simulink model "ICare_Simulink_Demo"  (R2026a)
settings: Solver=FixedStepDiscrete  StopTime=0
settings Model: Creator=ragav  LastModifiedBy=ragav

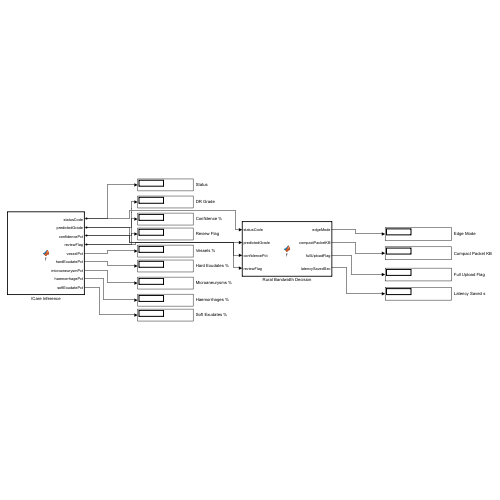
[thumbnail: Simulink's stored preview of the top-level diagram]
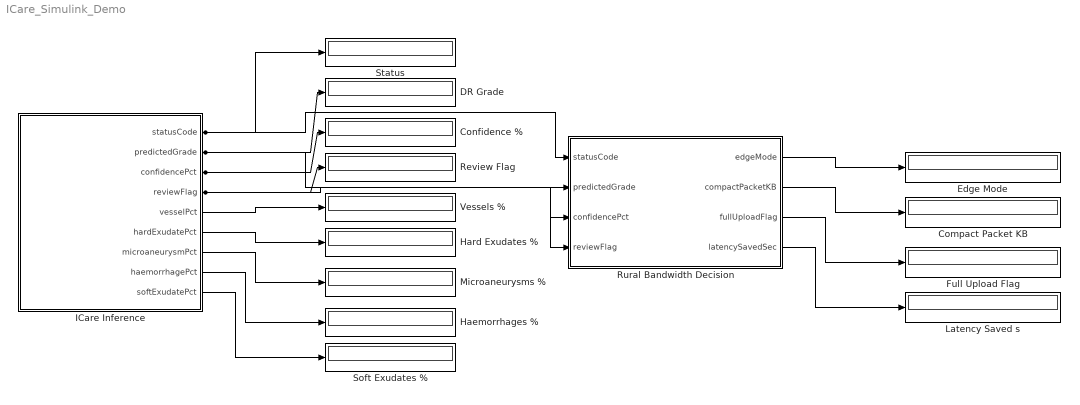
== system ICare_Simulink_Demo ==
  Compact Packet KB : Display
  Confidence % : Display
  DR Grade : Display
  Edge Mode : Display
  Full Upload Flag : Display
  Haemorrhages % : Display
  Hard Exudates % : Display
  ICare Inference : MATLAB Function  TreatAsAtomicUnit=on
  Latency Saved s : Display
  Microaneurysms % : Display
  Review Flag : Display
  Rural Bandwidth Decision : MATLAB Function  TreatAsAtomicUnit=on
  Soft Exudates % : Display
  Status : Display
  Vessels % : Display
  wires:
  ICare Inference/1(statusCode) -> Status/1, Rural Bandwidth Decision/1(statusCode)
  ICare Inference/2(predictedGrade) -> DR Grade/1, Rural Bandwidth Decision/2(predictedGrade)
  ICare Inference/3(confidencePct) -> Confidence %/1, Rural Bandwidth Decision/3(confidencePct)
  ICare Inference/4(reviewFlag) -> Review Flag/1, Rural Bandwidth Decision/4(reviewFlag)
  ICare Inference/5(vesselPct) -> Vessels %/1
  ICare Inference/6(hardExudatePct) -> Hard Exudates %/1
  ICare Inference/7(microaneurysmPct) -> Microaneurysms %/1
  ICare Inference/8(haemorrhagePct) -> Haemorrhages %/1
  ICare Inference/9(softExudatePct) -> Soft Exudates %/1
  Rural Bandwidth Decision/1(edgeMode) -> Edge Mode/1
  Rural Bandwidth Decision/2(compactPacketKB) -> Compact Packet KB/1
  Rural Bandwidth Decision/3(fullUploadFlag) -> Full Upload Flag/1
  Rural Bandwidth Decision/4(latencySavedSec) -> Latency Saved s/1

== matlab function ICare_Simulink_Demo/Rural Bandwidth Decision ==
  data: statusCode input; edgeMode output; predictedGrade input; confidencePct input; reviewFlag input; compactPacketKB output; fullUploadFlag output; latencySavedSec output
function [edgeMode, compactPacketKB, fullUploadFlag, latencySavedSec] = f(statusCode, predictedGrade, confidencePct, reviewFlag)
%%#codegen
% Rural screening assumption: low bandwidth link at the camp.
fullImageKB = 4096;
compactPacketKB = 12;
bandwidthKbps = 256;
cloudRoundTripSec = 3;
if statusCode < 1
    edgeMode = 0;
    fullUploadFlag = 0;
    latencySavedSec = 0;
    return;
end
highRisk = predictedGrade >= 2 || confidencePct < 50 || reviewFlag >= 1;
if highRisk
    edgeMode = 2;
    fullUploadFlag = 1;
else
    edgeMode = 1;
    fullUploadFlag = 0;
end
fullUploadSec = 8 * fullImageKB / bandwidthKbps + cloudRoundTripSec;
compactUploadSec = 8 * compactPacketKB / bandwidthKbps + cloudRoundTripSec;
latencySavedSec = fullUploadSec - compactUploadSec;
end

== matlab function ICare_Simulink_Demo/ICare Inference ==
  data: statusCode output; predictedGrade output; confidencePct output; reviewFlag output; vesselPct output; hardExudatePct output; microaneurysmPct output; haemorrhagePct output; softExudatePct output
function [statusCode, predictedGrade, confidencePct, reviewFlag, vesselPct, hardExudatePct, microaneurysmPct, haemorrhagePct, softExudatePct] = f()
%#codegen
coder.extrinsic('icare_simulink_predict');
statusCode = 0;
predictedGrade = -1;
confidence = 0;
reviewFlag = 1;
vesselFraction = NaN;
hardExudateFraction = NaN;
microaneurysmFraction = NaN;
haemorrhageFraction = NaN;
softExudateFraction = NaN;
[statusCode, predictedGrade, confidence, reviewFlag, vesselFraction, hardExudateFraction, microaneurysmFraction, haemorrhageFraction, softExudateFraction] = icare_simulink_predict('C:\Users\ragav\MATLAB Drive\ICare\data\APTOS\train_images\000c1434d8d7.png');
confidencePct = 100 * confidence;
vesselPct = 100 * vesselFraction;
hardExudatePct = 100 * hardExudateFraction;
microaneurysmPct = 100 * microaneurysmFraction;
haemorrhagePct = 100 * haemorrhageFraction;
softExudatePct = 100 * softExudateFraction;
end
